simulink model "untitled"  (R2022a)
settings: Solver=VariableStepAuto  StartTime=0.0  StopTime=10.0  RelTol=1e-3
undefined symbols (not defined in the file): A, B, C
settings Model: DataDictionary=test11.sldd  Creator=khari  LastModifiedBy=khari

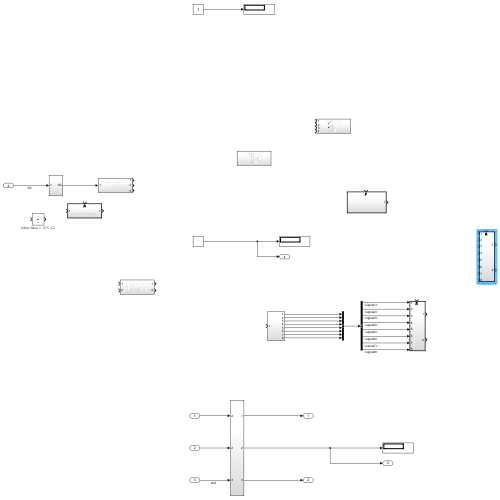
[thumbnail: Simulink's stored preview of the top-level diagram]
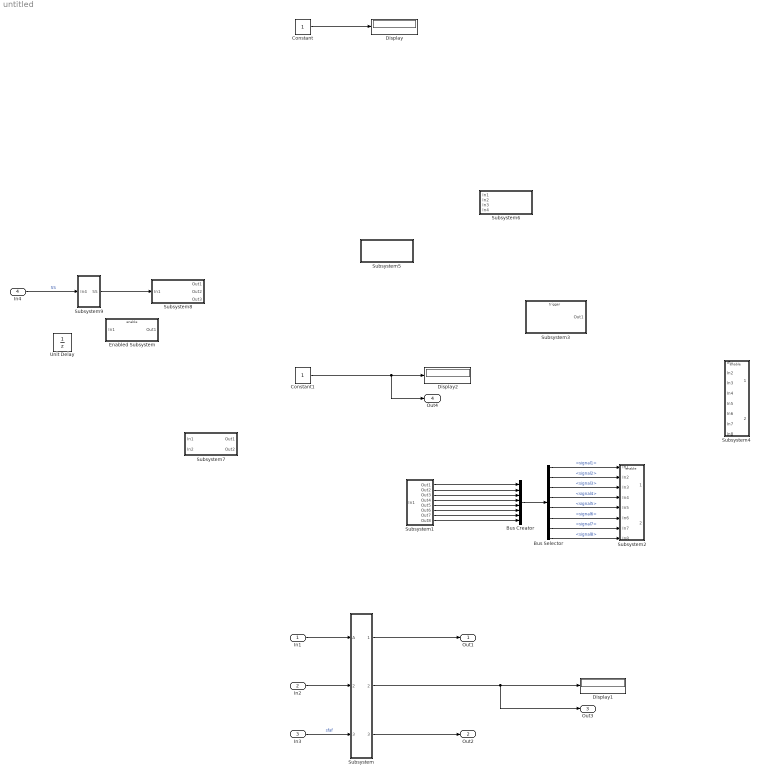
== system untitled ==
  In1 : Inport
  In2 : Inport  Port=2
  In3 : Inport  Port=3
  In4 : Inport  Port=4
  Bus Creator : BusCreator  Inputs=8
  Bus Selector : BusSelector  OutputSignals=signal1,signal2,signal3,signal4,signal5,signal6,signal7,signal8
  Constant : Constant
  Constant1 : Constant
  Display : Display
  Display1 : Display
  Display2 : Display
  Enabled Subsystem : Subsystem  TreatAsAtomicUnit=on
  Subsystem : Subsystem
  Subsystem1 : Subsystem
  Subsystem2 : Subsystem
  Subsystem3 : Subsystem
  Subsystem4 : Subsystem
  Subsystem5 : Subsystem
  Subsystem6 : Subsystem
  Subsystem7 : Subsystem
  Subsystem8 : Subsystem
  Subsystem9 : Subsystem
  Unit Delay : UnitDelay  InitialCondition=C  SampleTime=-1  HasFrameUpgradeWarning=on
      settings: AttributesFormatString=Initial Value = 12°C (C)
  Out1 : Outport
  Out2 : Outport  Port=2
  Out3 : Outport  Port=3
  Out4 : Outport  Port=4
  wires:
  Constant/1 -> Display/1
  Subsystem/2(Out3) -> Display1/1, Out3/1
  In1/1 -> Subsystem/1(A)
  In3/1 -> Subsystem/3(In3)  "sfaf"
  Subsystem/1(Out1) -> Out1/1
  Subsystem/3(Out2) -> Out2/1
  Subsystem1/2(Out2) -> Bus Creator/2
  Subsystem1/3(Out3) -> Bus Creator/3
  Subsystem1/1(Out1) -> Bus Creator/1
  Subsystem1/4(Out4) -> Bus Creator/4
  Subsystem1/5(Out5) -> Bus Creator/5
  Subsystem1/6(Out6) -> Bus Creator/6
  Subsystem1/7(Out7) -> Bus Creator/7
  Subsystem1/8(Out8) -> Bus Creator/8
  Bus Creator/1 -> Bus Selector/1
  Bus Selector/1 -> Subsystem2/1(In1)  "<signal1>"
  Bus Selector/2 -> Subsystem2/2(In2)  "<signal2>"
  Bus Selector/3 -> Subsystem2/3(In3)  "<signal3>"
  Bus Selector/4 -> Subsystem2/4(In4)  "<signal4>"
  Bus Selector/5 -> Subsystem2/5(In5)  "<signal5>"
  Bus Selector/6 -> Subsystem2/6(In6)  "<signal6>"
  Bus Selector/7 -> Subsystem2/7(In7)  "<signal7>"
  Bus Selector/8 -> Subsystem2/8(In8)  "<signal8>"
  Constant1/1 -> Display2/1, Out4/1
  In2/1 -> Subsystem/2(In2)
  In4/1 -> Subsystem9/1(In4)  "SS"
  Subsystem9/1(SS) -> Subsystem8/1(In1)

== system untitled/Enabled Subsystem ==
  In1 : Inport
  Enable : EnablePort
  Out1 : Outport  InitialOutput=C
      settings: AttributesFormatString=Init Value = 12°C (C)
  wires:
  In1/1 -> Out1/1

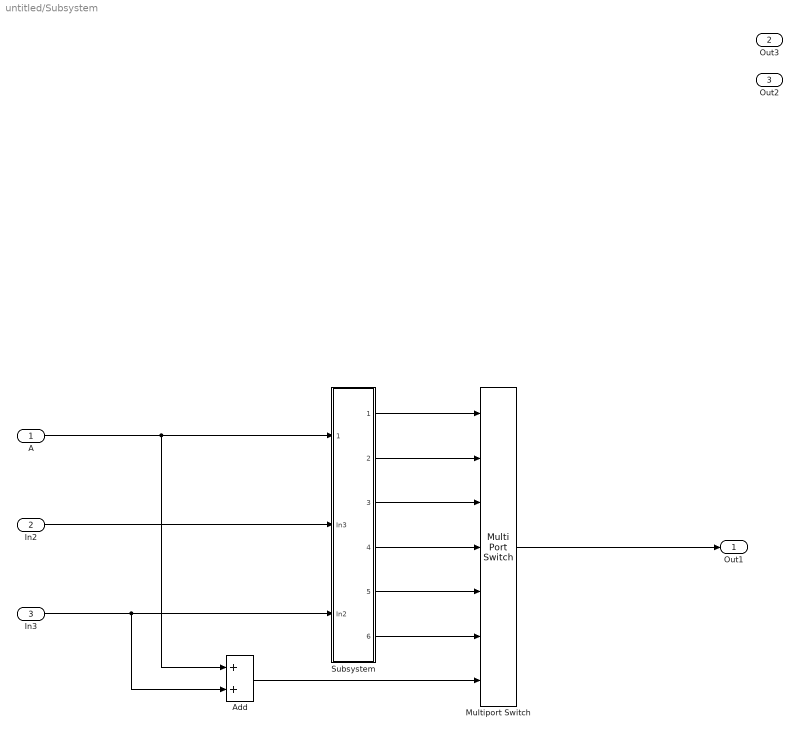
== system untitled/Subsystem ==
  A : Inport
  In2 : Inport  Port=2
  In3 : Inport  Port=3
  Add : Sum
  Multiport Switch : MultiPortSwitch  Inputs=6  SaturateOnIntegerOverflow=off  InputSameDT=off
  Subsystem : Subsystem
  Out1 : Outport
  Out3 : Outport  Port=2
  Out2 : Outport  Port=3
  wires:
  Multiport Switch/1 -> Out1/1
  A/1 -> Add/1, Subsystem/1(PI_Tnk3)
  In3/1 -> Add/2, Subsystem/3(In2)
  Subsystem/3(Tnk3) -> Multiport Switch/3
  Subsystem/2(Out2) -> Multiport Switch/2
  Subsystem/4(Out3) -> Multiport Switch/4
  Subsystem/6(Out4) -> Multiport Switch/6
  Subsystem/1(Out5) -> Multiport Switch/1
  In2/1 -> Subsystem/2(In3)
  Add/1 -> Multiport Switch/7
  Subsystem/5(Out6) -> Multiport Switch/5

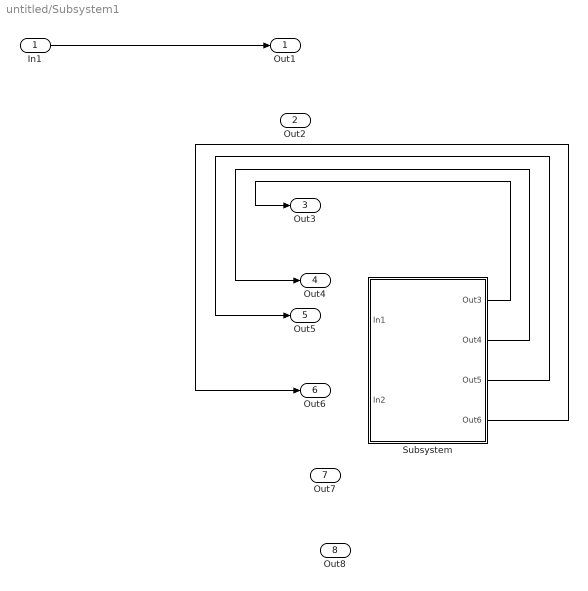
== system untitled/Subsystem1 ==
  In1 : Inport
  Subsystem : Subsystem
  Out1 : Outport
  Out2 : Outport  Port=2
  Out3 : Outport  Port=3
  Out4 : Outport  Port=4
  Out5 : Outport  Port=5
  Out6 : Outport  Port=6
  Out7 : Outport  Port=7
  Out8 : Outport  Port=8
  wires:
  In1/1 -> Out1/1
  ? -> Out7/1
  Subsystem/1(Out3) -> Out3/1
  Subsystem/2(Out4) -> Out4/1
  Subsystem/3(Out5) -> Out5/1
  Subsystem/4(Out6) -> Out6/1

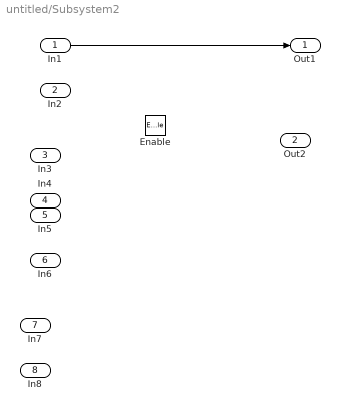
== system untitled/Subsystem2 ==
  In1 : Inport
  In2 : Inport  Port=2
  In3 : Inport  Port=3
  In4 : Inport  Port=4
  In5 : Inport  Port=5
  In6 : Inport  Port=6
  In7 : Inport  Port=7
  In8 : Inport  Port=8
  Enable : EnablePort
  Out1 : Outport  InitialOutput=A
      settings: AttributesFormatString=Init Value = 12 (A)
  Out2 : Outport  Port=2  InitialOutput=3
      settings: AttributesFormatString=Init Value = 3 (3)
  wires:
  In1/1 -> Out1/1

== system untitled/Subsystem3 ==
  Trigger : TriggerPort  VariantControl=(inherit)  PortDimensions=1
  Constant : Constant  Value=A
      settings: AttributesFormatString=Value = 12
  Constant1 : Constant  Value=B
  Out1 : Outport  InitialOutput=A
      settings: AttributesFormatString=Init Value = 12 (A)

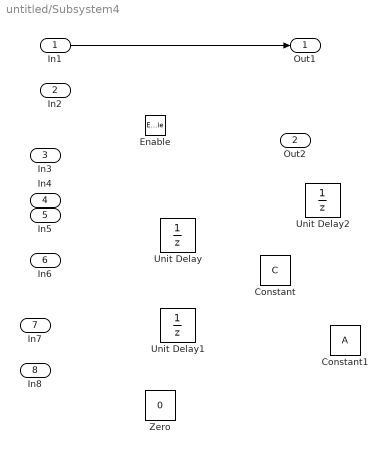
== system untitled/Subsystem4 ==
  In1 : Inport
  In2 : Inport  Port=2
  In3 : Inport  Port=3
  In4 : Inport  Port=4
  In5 : Inport  Port=5
  In6 : Inport  Port=6
  In7 : Inport  Port=7
  In8 : Inport  Port=8
  Enable : EnablePort
  Constant : Constant  Description=Hellp  Value=C
      settings: AttributesFormatString=Value = 12°C
  Constant1 : Constant  Description=Hellp  Value=A
      settings: AttributesFormatString=Value = 12
  Unit Delay : UnitDelay  InitialCondition=A  SampleTime=-1  HasFrameUpgradeWarning=on
      settings: AttributesFormatString=Initial Value = 12 (A)
  Unit Delay1 : UnitDelay  InitialCondition=C  SampleTime=-1  HasFrameUpgradeWarning=on
      settings: AttributesFormatString=Initial Value = 12°C (C)
  Unit Delay2 : UnitDelay  InitialCondition=C  SampleTime=-1  HasFrameUpgradeWarning=on
      settings: AttributesFormatString=Initial Value = 12°C (C)
  Zero : Constant  Value=0  OutDataTypeStr=Inherit: Inherit via back propagation
  Out1 : Outport  InitialOutput=C
      settings: AttributesFormatString=Init Value = 12°C (C)
  Out2 : Outport  Port=2  InitialOutput=3
      settings: AttributesFormatString=Init Value = 3 (3)
  wires:
  In1/1 -> Out1/1

== system untitled/Subsystem5 ==
  Subsystem : Subsystem
  Subsystem1 : Subsystem
  Subsystem2 : Subsystem
  Subsystem3 : Subsystem
  wires:
  Subsystem/1(Out1) -> Subsystem1/1(In1), Subsystem2/1(In1), Subsystem3/1(In1)
  Subsystem/2(Out2) -> Subsystem1/2(In2), Subsystem2/2(In2), Subsystem3/2(In2)
  Subsystem/3(Out3) -> Subsystem1/3(In3), Subsystem2/3(In3), Subsystem3/3(In3)
  Subsystem/4(Out4) -> Subsystem1/4(In4), Subsystem2/4(In4), Subsystem3/4(In4)

== system untitled/Subsystem6 ==
  In1 : Inport
  In2 : Inport  Port=2
  In3 : Inport  Port=3
  In4 : Inport  Port=4
  Subsystem1 : Subsystem
  Subsystem2 : Subsystem
  Subsystem3 : Subsystem
  wires:
  In1/1 -> Subsystem1/1(In1), Subsystem2/1(In1), Subsystem3/1(In1)
  In2/1 -> Subsystem1/2(In2), Subsystem2/2(In2), Subsystem3/2(In2)
  In3/1 -> Subsystem1/3(In3), Subsystem2/3(In3), Subsystem3/3(In3)
  In4/1 -> Subsystem1/4(In4), Subsystem2/4(In4), Subsystem3/4(In4)

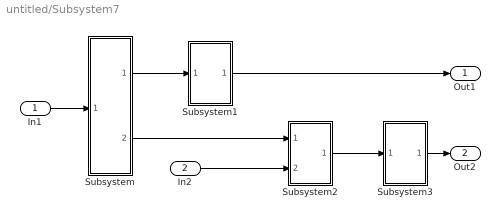
== system untitled/Subsystem7 ==
  In1 : Inport
  In2 : Inport  Port=2
  Subsystem : Subsystem
  Subsystem1 : Subsystem
  Subsystem2 : Subsystem
  Subsystem3 : Subsystem
  Out1 : Outport
  Out2 : Outport  Port=2
  wires:
  In1/1 -> Subsystem/1(In1)
  Subsystem/1(Out1) -> Subsystem1/1(In1)
  Subsystem1/1(Out1) -> Out1/1
  In2/1 -> Subsystem2/2(In2)
  Subsystem2/1(Out1) -> Subsystem3/1(In1)
  Subsystem3/1(Out2) -> Out2/1
  Subsystem/2(Out2) -> Subsystem2/1(In1)

== system untitled/Subsystem8 ==
  In1 : Inport
  Gain : Gain
  Gain1 : Gain
  Out1 : Outport
  Out2 : Outport  Port=2
  Out3 : Outport  Port=3
  wires:
  In1/1 -> Gain/1
  Gain/1 -> Out2/1, Gain1/1  "IntermediateSignal"
  Gain1/1 -> Out1/1  "OutputSig1"

== system untitled/Subsystem9 ==
  In4 : Inport
  SS : Outport
  wires:
  In4/1 -> SS/1

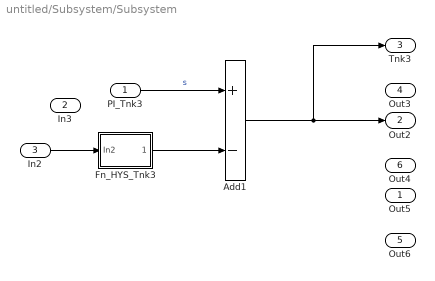
== system untitled/Subsystem/Subsystem ==
  PI_Tnk3 : Inport
  In3 : Inport  Port=2
  In2 : Inport  Port=3
  Add1 : Sum  Inputs=+-
  Fn_HYS_Tnk3 : Subsystem
  Out5 : Outport
  Out2 : Outport  Port=2
  Tnk3 : Outport  Port=3
  Out3 : Outport  Port=4
  Out6 : Outport  Port=5
  Out4 : Outport  Port=6
  wires:
  PI_Tnk3/1 -> Add1/1  "s"
  Add1/1 -> Tnk3/1, Out2/1
  In2/1 -> Fn_HYS_Tnk3/1(In2)
  Fn_HYS_Tnk3/1(PO_HYS_Tnk3) -> Add1/2

== system untitled/Subsystem1/Subsystem ==
  In1 : Inport
  In2 : Inport  Port=2
  Out3 : Outport
  Out4 : Outport  Port=2
  Out5 : Outport  Port=3
  Out6 : Outport  Port=4
  wires:
  In1/1 -> Out3/1
  In2/1 -> Out5/1

== system untitled/Subsystem5/Subsystem ==
  In1 : Inport
  Out1 : Outport
  Out2 : Outport  Port=2
  Out3 : Outport  Port=3
  Out4 : Outport  Port=4
  wires:
  In1/1 -> Out1/1

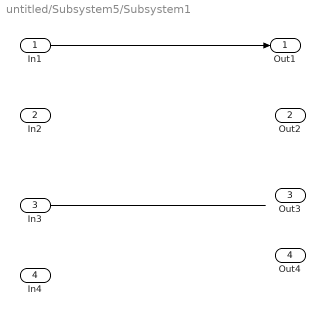
== system untitled/Subsystem5/Subsystem1 ==
  In1 : Inport
  In2 : Inport  Port=2
  In3 : Inport  Port=3
  In4 : Inport  Port=4
  Out1 : Outport
  Out2 : Outport  Port=2
  Out3 : Outport  Port=3
  Out4 : Outport  Port=4
  wires:
  In1/1 -> Out1/1
  In3/1 -> ?

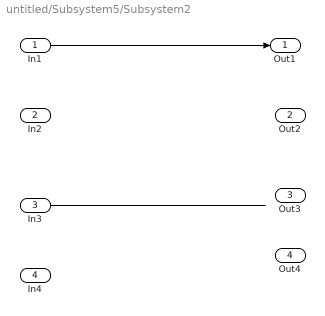
== system untitled/Subsystem5/Subsystem2 ==
  In1 : Inport
  In2 : Inport  Port=2
  In3 : Inport  Port=3
  In4 : Inport  Port=4
  Out1 : Outport
  Out2 : Outport  Port=2
  Out3 : Outport  Port=3
  Out4 : Outport  Port=4
  wires:
  In3/1 -> ?
  In1/1 -> Out1/1

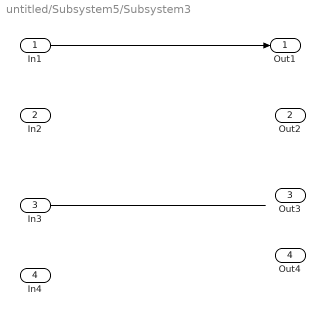
== system untitled/Subsystem5/Subsystem3 ==
  In1 : Inport
  In2 : Inport  Port=2
  In3 : Inport  Port=3
  In4 : Inport  Port=4
  Out1 : Outport
  Out2 : Outport  Port=2
  Out3 : Outport  Port=3
  Out4 : Outport  Port=4
  wires:
  In1/1 -> Out1/1
  In3/1 -> ?

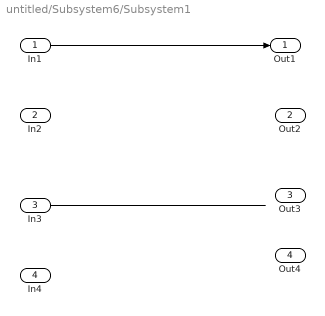
== system untitled/Subsystem6/Subsystem1 ==
  In1 : Inport
  In2 : Inport  Port=2
  In3 : Inport  Port=3
  In4 : Inport  Port=4
  Out1 : Outport
  Out2 : Outport  Port=2
  Out3 : Outport  Port=3
  Out4 : Outport  Port=4
  wires:
  In3/1 -> ?
  In1/1 -> Out1/1

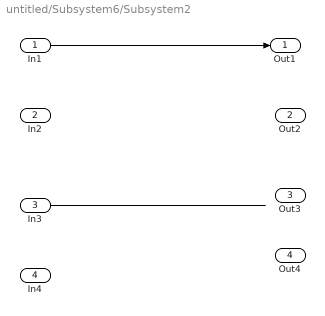
== system untitled/Subsystem6/Subsystem2 ==
  In1 : Inport
  In2 : Inport  Port=2
  In3 : Inport  Port=3
  In4 : Inport  Port=4
  Out1 : Outport
  Out2 : Outport  Port=2
  Out3 : Outport  Port=3
  Out4 : Outport  Port=4
  wires:
  In1/1 -> Out1/1
  In3/1 -> ?

== system untitled/Subsystem6/Subsystem3 ==
  In1 : Inport
  In2 : Inport  Port=2
  In3 : Inport  Port=3
  In4 : Inport  Port=4
  Out1 : Outport
  Out2 : Outport  Port=2
  Out3 : Outport  Port=3
  Out4 : Outport  Port=4
  wires:
  In3/1 -> ?
  In1/1 -> Out1/1

== system untitled/Subsystem7/Subsystem ==
  In1 : Inport
  Out1 : Outport
  Out2 : Outport  Port=2
  wires:
  In1/1 -> Out1/1

== system untitled/Subsystem7/Subsystem1 ==
  In1 : Inport
  Out1 : Outport
  wires:
  In1/1 -> Out1/1

== system untitled/Subsystem7/Subsystem2 ==
  In1 : Inport
  In2 : Inport  Port=2
  Out1 : Outport
  wires:
  In2/1 -> Out1/1

== system untitled/Subsystem7/Subsystem3 ==
  In1 : Inport
  Out2 : Outport
  wires:
  In1/1 -> Out2/1

== system untitled/Subsystem/Subsystem/Fn_HYS_Tnk3 ==
  In2 : Inport
  PO_HYS_Tnk3 : Outport
  wires:
  In2/1 -> PO_HYS_Tnk3/1
